simulink model "S_MPPT_ALGS_PIL_SIM_V1"  (R2017a)
settings: Solver=VariableStepAuto  StartTime=0.0  StopTime=5  FixedStep=1e-6  MaxStep=1e-4  RelTol=1e-3
values from neighbouring files (symbols this model uses):
  Alpha1 = 2*Zeta_obs*wn_obs    (= 2)    [M_MPPT_ALGS_PIL_SIM_V1.m]
  Alpha2 = wn_obs    (= 1)    [M_MPPT_ALGS_PIL_SIM_V1.m]
  Cdc = Cdc    (= 0.00047)    [M_MPPT_ALGS_PIL_SIM_V1.m]
  Cpv = Cpv    (= 8e-05)    [M_MPPT_ALGS_PIL_SIM_V1.m]
  Epsilon = Ep_cont/Ts1    [M_MPPT_ALGS_PIL_SIM_V1.m]
  ESRCdc = ESRCdc    (= 0.2)    [M_MPPT_ALGS_PIL_SIM_V1.m]
  ESRCpv = ESRCpv    (= 0.2)    [M_MPPT_ALGS_PIL_SIM_V1.m]
  Fred = fs    (= 60)    [M_MPPT_ALGS_PIL_SIM_V1.m]
  fs = 60    [M_MPPT_ALGS_PIL_SIM_V1.m]
  G_STC = 1000    [M_MPPT_ALGS_PIL_SIM_V1.m]
  Icc_calc = In/(5/100)    [M_MPPT_ALGS_PIL_SIM_V1.m]
  impp_STC = 15.72/2    (= 7.86)    [M_MPPT_ALGS_PIL_SIM_V1.m]
  K1 = Kt_acker_d    [M_MPPT_ALGS_PIL_SIM_V1.m]
  K1y2md = Kmd(1:end-1)    [M_MPPT_ALGS_PIL_SIM_V1.m]
  Kdpwm = 1/Ucmax    (= 1.52590218967e-05)    [M_MPPT_ALGS_PIL_SIM_V1.m]
  KI1 = Kp1/Ti1*Ts1    (= 1900)    [M_MPPT_ALGS_PIL_SIM_V1.m]
  KI2 = Ki2*Ts4    [M_MPPT_ALGS_PIL_SIM_V1.m]
  KI4 = Ki4*Ts4    [M_MPPT_ALGS_PIL_SIM_V1.m]
  KI5 = Ki5*Ts_inv    (= 0.17765287922)    [M_MPPT_ALGS_PIL_SIM_V1.m]
  Kimd = -Kmd(end)    [M_MPPT_ALGS_PIL_SIM_V1.m]
  KP1 = Kp1-KI1/2    (= 21850)    [M_MPPT_ALGS_PIL_SIM_V1.m]
  KP2 = Kp2-KI2/2    [M_MPPT_ALGS_PIL_SIM_V1.m]
  KP4 = Kp4-KI4/2    [M_MPPT_ALGS_PIL_SIM_V1.m]
  KP5 = Kp5*Ts_inv-KI5/2    (= -0.0874937760062)    [M_MPPT_ALGS_PIL_SIM_V1.m]
  L = L    (= 0.1)    [M_MPPT_ALGS_PIL_SIM_V1.m]
  Linv = 0.03    [M_MPPT_ALGS_PIL_SIM_V1.m]
  Npar = No_Cadenas_Paralelo    (= 2)    [M_MPPT_ALGS_PIL_SIM_V1.m]
  Rinv = 0.0417    [M_MPPT_ALGS_PIL_SIM_V1.m]
  RL = RL    (= 0.3)    [M_MPPT_ALGS_PIL_SIM_V1.m]
  S = 10e3*3/2    (= 15000)    [M_MPPT_ALGS_PIL_SIM_V1.m]
  Ts = Ts1    (= 0.0002)    [M_MPPT_ALGS_PIL_SIM_V1.m]
  Ts1 = 1/Fs    (= 0.0002)    [M_MPPT_ALGS_PIL_SIM_V1.m]
  Ts4 = 1/(4*Fc)    (= 0.000125)    [M_MPPT_ALGS_PIL_SIM_V1.m]
  Ts_inv = 1/(100*Fc)    (= 5e-06)    [M_MPPT_ALGS_PIL_SIM_V1.m]
  Ucmax = (2^b-1)    (= 65535)    [M_MPPT_ALGS_PIL_SIM_V1.m]
  vdc = 1000    [M_MPPT_ALGS_PIL_SIM_V1.m]
  vdc_ref = vdc    (= 1000)    [M_MPPT_ALGS_PIL_SIM_V1.m]
  Vf = VL/sqrt(3)    [M_MPPT_ALGS_PIL_SIM_V1.m]
  VL = (381.051/2)    (= 190.5255)    [M_MPPT_ALGS_PIL_SIM_V1.m]
undefined symbols (not defined in the file or in its folder): DiscIntNeverNeededParam
undefined symbols (not defined in the file): Fs
libraries: powerlib x15, powerlib_meascontrol x12, dsparch4 x3, re_lib x1
(part 1 of 2)
settings Model: ExtModeTrigDuration=10  Creator=dricl  LastModifiedBy=dricl
settings OptimizationCC: PassReuseOutputArgsAs=Individual arguments  MaxStackSize=2560
settings DebuggingCC: ParameterTunabilityLossMsg=error
settings HardwareCC: ProdBitPerPointer=32  ProdBitPerSizeT=32  ProdBitPerPtrDiffT=32  ProdLargestAtomicInteger=Long  ProdLargestAtomicFloat=Double  ProdWordSize=32  ProdLongLongMode=on  ProdHWDeviceType=ARM Compatible->ARM Cortex
settings SFSimCC: MATLABDynamicMemAlloc=off
settings RTWCC: SystemTargetFile=ert.tlc  HardwareBoard=TI Concerto F28M35x (ARM Cortex-M3)  TLCOptions=-aInlineSetEventsForThisBaseRateFcn=TLC_FALSE -aSuppressMultiTaskScheduler=TLC_FALSE -aRateBasedStepFcn=1  TemplateMakefile=ert_default_tmf  Description=Embedded Coder  GenerateReport=on  Toolchain=Texas Instruments Code Composer Studio v6 (ARM)  IncludeHyperlinkInReport=on  LaunchReport=on  CreateSILPILBlock=PIL  GenerateTraceInfo=on  GenerateTraceReport=on  GenerateTraceReportSl=on  GenerateTraceReportSf=on  GenerateTraceReportEml=on
settings CodeAppCC: ForceParamTrailComments=on  IgnoreCustomStorageClasses=off  OperatorAnnotations=on  SimulinkDataObjDesc=on  SFDataObjDesc=on  MATLABFcnDesc=on  InsertBlockDesc=on  MATLABSourceComments=on

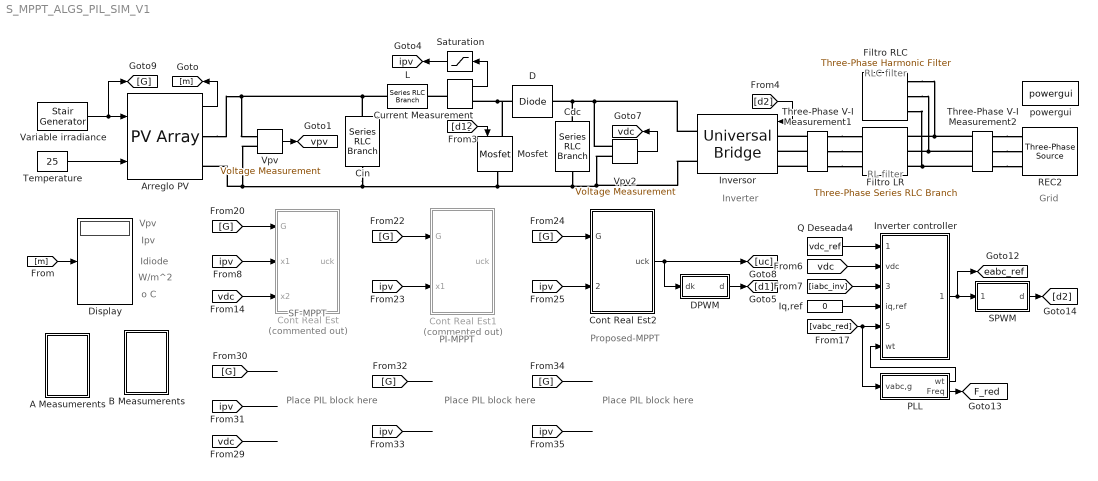
== system S_MPPT_ALGS_PIL_SIM_V1 ==
  note: Grid
  note: W/m^2
  note: Idiode
  note: Vpv
  note: RLC filter
  note: Ipv
  note: SF-MPPT
  note: PI-MPPT
  note: o C
  note: Proposed-MPPT
  note: RL filter
  note: Inverter
  note: Place PIL
      | block here
  note: Place PIL
      | block here
  note: Place PIL
      | block here
  " Variable irradiance" : powerlib_meascontrol/Pulse & Signal Generators/Stair Generator  t=[0, 0.1, 0.3, 0.5, 0.7, 0.8, 0.9, 1.0, 1.1, 1.2, 1.3, 1.4, 1.5, 1.6, 1.7, 1.8, 1.9, 2.0, 2.1, 2.2, 2.3, 2.4, 2.5, 2.6, 2.7, 2.8, 2.9, 3.0, 3.1, 3.2, 3.3, 3.4, 3.5, 3.6, 3.7, 3.8, 3.9, 4.0, 4.1, 4.2, 4.3, 4.4, 4.5, 4.6, 4.7, 4.8, 4.9, 5.0]  e=[0, 1000, 400, 900, 607.1, 607.1, 652.7, 685.8, 715.6, 742.3, 765.3, 795, 812, 840, 839, 893, 596.3, 420.8, 1037, 974, 948, 921, 970, 985, 991, 700, 1004, 997, 993, 1001, 998, 1033, 656.5, 1027, 954, 938, 937, 906, 705.4, 860, 773, 670.6, 450.3, 409.6, 682.2, 639.9, 601, 415.5]  Ts=0
      settings: SourceProductName=Simscape Power Systems
  A Measumerents : Subsystem
  Arreglo PV : re_lib/Solar/PV Array  Npar=No_Cadenas_Paralelo  Nser=No_Modulos_PorCadena  PlotType=array @ 25 deg.C & specified irradiances  S_vec=[1037]  Temp_C_vec="[ 45 25  0]"  ModuleName=Canadian Solar CS6X-280P  PlotWhenSelected=off  Pm=279.816  Ncell=72  Voc=44.2  Isc=8.42  Vm=35.6  Im=7.86  beta_Voc_pc=-0.39  alpha_Isc_pc=0.06  beta_Voc=-0.17238  alpha_Isc=0.005052  IL=8.4417  I0=7.7188e-10  nI=1.0345  Rsh=300.2269  Rs=0.38773  BAL=off  Tc=1e-6  Tfilter=5e-5
  B Measumerents : Subsystem
  Cdc : powerlib/Elements/Series RLC Branch  LConnTagsString=__new0  RConnTagsString=__new0  BranchType=RC  Resistance=ESRCdc  Inductance=1e-3  SetiL0=off  InitialCurrent=0  Capacitance=Cdc  Setx0=on  InitialVoltage=vdc_ref  Measurements=None
  Cin : powerlib/Elements/Series RLC Branch  LConnTagsString=__new0  RConnTagsString=__new0  BranchType=RC  Resistance=ESRCpv  Inductance=1e-3  SetiL0=off  InitialCurrent=0  Capacitance=Cpv  Setx0=off  InitialVoltage=640.8  Measurements=None
  Cont Real Est : Subsystem  Commented=on
  Cont Real Est1 : Subsystem  Commented=on
  Cont Real Est2 : Subsystem
  Current Measurement2 : powerlib/Measurements/Current Measurement  PhasorSimulation=off  OutputType=Complex  PSBequivalent=0
  D : powerlib/Power Electronics/Diode  Ron=Rondiode  Lon=0  Vf=Vfdiode  IC=0  UseSnubber=0  Rs=500  Cs=250e-9  Measurements=off
  DPWM : Subsystem  AncestorBlock=plecslib_extras2/Modulators/Symmetrical PWM  mask(Symmetrical PWM){sampling=Natural (carrier starts with 0), fc=Fs, offset=0, input_limits=[0 Ucmax], output_values=[0 1]}
      mask prompts: fc "Carrier frequency (Hz):"; offset "Carrier offset (p.u.):"; input_limits "Input limits [min max]:"; output_values "Output values [off on]:"
      mask help: PWM generator with a symmetrical triangular carrier. If the input is a vector, the output is also a vector of the same width.
      mask init:
      | if numel(fc)>1 || fc<=0,
      |   error('Carrier frequency must be a positive scalar.');
      | end
      | if numel(offset)>1 || offset<0 || offset>=1,
      |   error('Carrier offset must be a scalar in the range [0; 1/fc[.');
      | end
      | if sampling == 1,
      |   offset = mod(offset+.75, 1);
      | end
      | 
      | si = [.5 mod(offset, .5)]/fc;
      mask Help: eval('plecs(''help'', ''symmetricalpwm.html'')')
      mask TypeOptions sampling: Natural (carrier starts with 0) | Natural (carrier starts with 1) | Regular (double edge) | Regular (single edge)
  Display : Display
  Filtro LR : powerlib/Elements/Three-Phase Series RLC Branch  LConnTagsString=A|B|C  RConnTagsString=A|B|C  BranchType=RL  Resistance=Rinv  Inductance=Linv  Capacitance=1e-6  Measurements=None
  Filtro RLC : powerlib/Elements/Three-Phase Harmonic Filter  LConnTagsString=A|B|C  FilterType=Single-tuned  FilterConnection=Y (grounded)  ParNom=[VL fs]  Qc=S*0.001  Fr=[31.42*60]  Frd=[40*fs 80*fs]  Q=5  Measurements=None
      settings: AttributesFormatString=\n  SourceProductName=Simscape Power Systems  SourceProductBaseCode=PS
  Inversor : powerlib/Power Electronics/Universal Bridge  Arms=3  SnubberResistance=1e5  SnubberCapacitance=inf  Device=IGBT / Diodes  Ron=1e-3  Lon=0  ForwardVoltages="[  0  0  ]"  ForwardVoltage=0  GTOparameters=[ 10e-6 , 20e-6 ]  IGBTparameters=[ 1e-6 , 2e-6 ]  Measurements=None  Measurements_2=None  converterType=Rectifier
  Inverter controller : Subsystem
  Iq,ref : Constant  Value=0  SampleTime=Ts4
  L : powerlib/Elements/Series RLC Branch  LConnTagsString=__new0  RConnTagsString=__new0  BranchType=RL  Resistance=RL  Inductance=L  SetiL0=off  InitialCurrent=0  Capacitance=1e-6  Setx0=off  InitialVoltage=0  Measurements=None
  Mosfet : powerlib/Power Electronics/Mosfet  Ron=Ronfet  Lon=0  Rd=0  Vfd=0  IC=0  Rs=1e5  Cs=inf  Measurements=off
  PLL : Subsystem
  Q Deseada4 : Constant  Value=vdc_ref  SampleTime=Ts4
  REC2 : powerlib/Electrical Sources/Three-Phase Source  InternalConnection=Yg  VoltagePhases=on  Voltage=VL  PhaseAngle=0  Voltage_phases=[VL/sqrt(3) VL/sqrt(3) VL/sqrt(3)]  PhaseAngles_phases=[0 -120 +120]  Frequency=Fred  NonIdealSource=on  SpecifyImpedance=on  Resistance=25e3^2/10e6/5  Inductance=25e3^2/10e6/377  ShortCircuitLevel=Icc_calc*2  BaseVoltage=VL  XRratio=7  BusType=swing  Pref=-500e3  Qref=0  Prefabc=[10e3, 10e3, 10e3]  Qrefabc=[0, 0, 0]  Qmin=-inf  Qmax=inf
  SPWM : Subsystem
  Saturation : Saturate  UpperLimit=inf  LowerLimit=0
  Temperature : Constant  Value=25
  Three-Phase V-I Measurement1 : powerlib/Measurements/Three-Phase V-I Measurement  VoltageMeasurement=phase-to-ground  SetLabelV=on  LabelV=vabc_inv  Vpu=off  VpuLL=off  CurrentMeasurement=yes  SetLabelI=on  LabelI=iabc_inv  Ipu=off  Pbase=100e6  Vbase=500e3  OutputType=Complex  PhasorSimulation=off  PSBequivalent=0
  Three-Phase V-I Measurement2 : powerlib/Measurements/Three-Phase V-I Measurement  VoltageMeasurement=phase-to-ground  SetLabelV=on  LabelV=vabc_red  Vpu=off  VpuLL=off  CurrentMeasurement=yes  SetLabelI=on  LabelI=iabc_red  Ipu=off  Pbase=100e6  Vbase=500e3  OutputType=Complex  PhasorSimulation=off  PSBequivalent=0
  Vpv : powerlib/Measurements/Voltage Measurement  PhasorSimulation=off  OutputType=Complex  PSBequivalent=0
  Vpv2 : powerlib/Measurements/Voltage Measurement  PhasorSimulation=off  OutputType=Complex  PSBequivalent=0
  powergui : powerlib/powergui  Priority=1  SimulationMode=Continuous  SampleTime=1e-6  frequency=60  Iterations=50  frequencyindice=0  Pbase=100e6  ErrMax=1e-4  UnitsV=kV  UnitsW=MW  buscounter=0  FunctionMessages=off  echomessages=off  EnableUseOfTLC=off  CurrentSourceSwitches=off  DisableSnubberDevices=off  DisableRonSwitches=off  DisableVfSwitches=off  DisplayEquations=off  SolverType=Tustin/Backward Euler (TBE)  Interpol=off  ExternalGateDelay=off  methode=off  Ts=100  x0status=blocks  SPID=on  SwTol=0  HookPort=off  RestoreLinks=warning  ResistiveCurrentMeasurement=off  Frange=[0:2:500]  Ylog=off  Xlog=on  ShowGrid=off  save=off  variable=ZData  structure=0  ZoomFFT=off  StartTime=0.0  cycles=1  DisplayStyle=1  fundamental=60  FreqAxis=off  MaxFrequency=1000  frequencyindicesteady=1  RmsSteady=1  display=off
  tag scope: F_red=global, eabc_ref=global, ipv=global, vdc=global, vpv=global
  wires:
  [iabc_inv] -> Inverter controller/3(iabc,inv)
  Iq,ref/1 -> Inverter controller/4(iq,ref)
  Vpv2/1 -> [vdc]
  Q Deseada4/1 -> Inverter controller/1(vdc,ref)
  PLL/2(Freq) -> [F_red]
  SPWM/1(d) -> [d2]
  DPWM/1(d) -> [d1]
  Saturation/1 -> [ipv]
  Temperature/1 -> Arreglo PV/2
  [vdc] -> Inverter controller/2(vdc)
  PLL/1(wt) -> Inverter controller/6(wt)
  [vabc_red] -> PLL/1(vabc,g), Inverter controller/5(vabc,red)
  [d2] -> Inversor/1
  Vpv/1 -> [vpv]
  Inverter controller/1(eabc,ref) -> SPWM/1(eabc,ref), [eabc_ref]
  [d1] -> Mosfet/1
  Current Measurement2/1 -> Saturation/1
  [m] -> Display/1
  Arreglo PV/1 -> [m]
  [G] -> Cont Real Est1/1(G)
  [ipv] -> Cont Real Est1/2(x1)
  [ipv] -> Cont Real Est2/2(x1 = ipv)
  [ipv] -> Cont Real Est/2(x1)
  [vdc] -> Cont Real Est/3(x2)
  [G] -> Cont Real Est/1(G)
  " Variable irradiance"/1 -> [G], Arreglo PV/1
  [G] -> Cont Real Est2/1(G)
  [G] -> ?
  [ipv] -> ?
  [G] -> ?
  [ipv] -> ?
  [G] -> ?
  [ipv] -> ?
  [vdc] -> ?
  Cont Real Est2/1(uck) -> DPWM/1(dk), [uc]
  connections:
  Arreglo PV/RConn1 -- L/LConn1 -- Cin/LConn1 -- Vpv/LConn1
  Filtro RLC/LConn1 -- Filtro LR/RConn1 -- Three-Phase V-I Measurement2/LConn1
  Three-Phase V-I Measurement2/RConn1 -- REC2/RConn1
  Cdc/RConn1 -- Inversor/RConn2 -- Vpv2/LConn2 -- Vpv/LConn2 -- Arreglo PV/RConn2 -- Cin/RConn1 -- Mosfet/RConn1
  Filtro RLC/LConn2 -- Filtro LR/RConn2 -- Three-Phase V-I Measurement2/LConn2
  Three-Phase V-I Measurement2/RConn2 -- REC2/RConn2
  D/RConn1 -- Cdc/LConn1 -- Vpv2/LConn1 -- Inversor/RConn1
  Filtro RLC/LConn3 -- Filtro LR/RConn3 -- Three-Phase V-I Measurement2/LConn3
  Three-Phase V-I Measurement2/RConn3 -- REC2/RConn3
  Current Measurement2/RConn1 -- D/LConn1 -- Mosfet/LConn1
  Three-Phase V-I Measurement1/RConn1 -- Filtro LR/LConn1
  Three-Phase V-I Measurement1/RConn2 -- Filtro LR/LConn2
  Three-Phase V-I Measurement1/RConn3 -- Filtro LR/LConn3
  Three-Phase V-I Measurement1/LConn2 -- Inversor/LConn2
  Current Measurement2/LConn1 -- L/RConn1
  Three-Phase V-I Measurement1/LConn1 -- Inversor/LConn1
  Three-Phase V-I Measurement1/LConn3 -- Inversor/LConn3

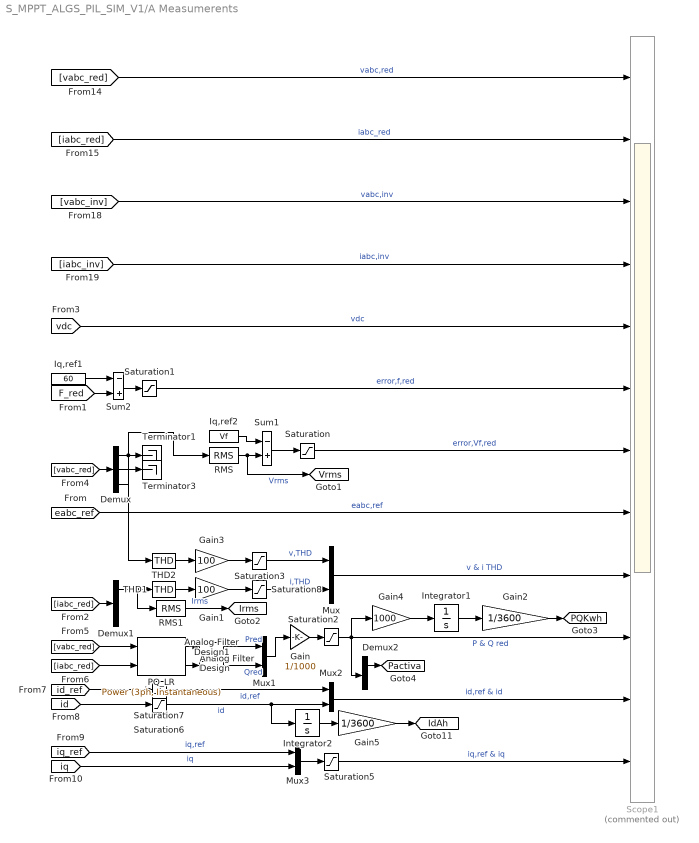
== system S_MPPT_ALGS_PIL_SIM_V1/A Measumerents ==
  Analog Filter Design : dsparch4/Analog Filter Design  method=Butterworth  filttype=Lowpass  N=8  Wlo=4000  Whi=80  Rp=2  Rs=40
  Analog Filter Design1 : dsparch4/Analog Filter Design  method=Butterworth  filttype=Lowpass  N=8  Wlo=4000  Whi=80  Rp=2  Rs=40
  Demux : Demux  Outputs=3
  Demux1 : Demux  Outputs=3
  Demux2 : Demux  Outputs=2
  Gain : Gain  Gain=1/1000
  Gain1 : Gain  Gain=100
  Gain2 : Gain  Gain=1/3600
  Gain3 : Gain  Gain=100
  Gain4 : Gain  Gain=1000
  Gain5 : Gain  Gain=1/3600
  Integrator1 : Integrator  ZeroCross=off
  Integrator2 : Integrator  ZeroCross=off
  Iq,ref1 : Constant  Value=60  SampleTime=Ts4
  Iq,ref2 : Constant  Value=Vf  SampleTime=Ts4
  Mux{,1..3} (4 alike) : Mux  Inputs=2
  PQ_LR : powerlib_meascontrol/Measurements/Power (3ph, Instantaneous)
      settings: SourceProductName=Simscape Power Systems
  RMS : powerlib_meascontrol/Measurements/RMS  TrueRMS=on  Freq=60  RMSInit=0  Ts=0
  RMS1 : powerlib_meascontrol/Measurements/RMS  TrueRMS=on  Freq=60  RMSInit=0  Ts=0
  Saturation : Saturate  UpperLimit=5.5  LowerLimit=-5.5
  Saturation1 : Saturate  UpperLimit=1  LowerLimit=-1
  Saturation2 : Saturate  UpperLimit=20  LowerLimit=0
  Saturation3 : Saturate  UpperLimit=20  LowerLimit=0
  Saturation5 : Saturate  UpperLimit=100  LowerLimit=0
  Saturation6 : Saturate  UpperLimit=inf  LowerLimit=0
  Saturation7 : Saturate  UpperLimit=inf  LowerLimit=0
  Saturation8 : Saturate  UpperLimit=20  LowerLimit=0
  Scope1 : Scope  Commented=on  NumInputPorts=12
  Sum1 : Sum  Inputs=-+
  Sum2 : Sum  Inputs=-+
  THD1 : powerlib_meascontrol/Measurements/THD  Freq=60  Ts=0
  THD2 : powerlib_meascontrol/Measurements/THD  Freq=60  Ts=0
  Terminator1 : Terminator
  Terminator3 : Terminator
  tag scope: IdAh=global, Irms=global, PQKwh=global, Pactiva=global, Vrms=global
  wires:
  Saturation/1 -> Scope1/7  "error,Vf,red"
  [vabc_red] -> Scope1/1  "vabc,red"
  [eabc_ref] -> Scope1/8  "eabc,ref"
  [iabc_red] -> Scope1/2  "iabc_red"
  Demux/1 -> THD2/1, RMS/1
  [vdc] -> Scope1/5  "vdc"
  [iabc_inv] -> Scope1/4  "iabc,inv"
  [vabc_inv] -> Scope1/3  "vabc,inv"
  Sum1/1 -> Saturation/1
  RMS/1 -> [Vrms], Sum1/2  "Vrms"
  Demux/2 -> Terminator3/1
  Demux/3 -> Terminator1/1
  [vabc_red] -> Demux/1
  [F_red] -> Sum2/2
  Iq,ref2/1 -> Sum1/1
  Iq,ref1/1 -> Sum2/1
  Saturation1/1 -> Scope1/6  "error,f,red"
  Sum2/1 -> Saturation1/1
  [iabc_red] -> Demux1/1
  Demux1/1 -> RMS1/1, THD1/1
  THD2/1 -> Gain3/1
  THD1/1 -> Gain1/1
  Mux/1 -> Scope1/9  "v & i THD"
  [vabc_red] -> PQ_LR/1
  [iabc_red] -> PQ_LR/2
  PQ_LR/1 -> Analog Filter Design/1
  Analog Filter Design/1 -> Mux1/1  "Pred"
  PQ_LR/2 -> Analog Filter Design1/1
  Analog Filter Design1/1 -> Mux1/2  "Qred"
  Saturation2/1 -> Demux2/1, Gain4/1, Scope1/10  "P & Q red"
  Gain/1 -> Saturation2/1
  Mux1/1 -> Gain/1
  Mux3/1 -> Saturation5/1
  [iq] -> Mux3/2  "iq"
  [id] -> Saturation6/1
  [iq_ref] -> Mux3/1  "iq,ref"
  [id_ref] -> Saturation7/1
  Mux2/1 -> Scope1/11  "id,ref & id"
  Saturation5/1 -> Scope1/12  "iq,ref & iq"
  RMS1/1 -> [Irms]  "Irms"
  Saturation6/1 -> Integrator2/1, Mux2/2  "id"
  Saturation7/1 -> Mux2/1  "id,ref"
  Gain3/1 -> Saturation3/1
  Saturation3/1 -> Mux/1  "v,THD"
  Saturation8/1 -> Mux/2  "i,THD"
  Gain1/1 -> Saturation8/1
  Integrator2/1 -> Gain5/1
  Integrator1/1 -> Gain2/1
  Demux2/1 -> [Pactiva]
  Gain2/1 -> [PQKwh]
  Gain4/1 -> Integrator1/1
  Gain5/1 -> [IdAh]

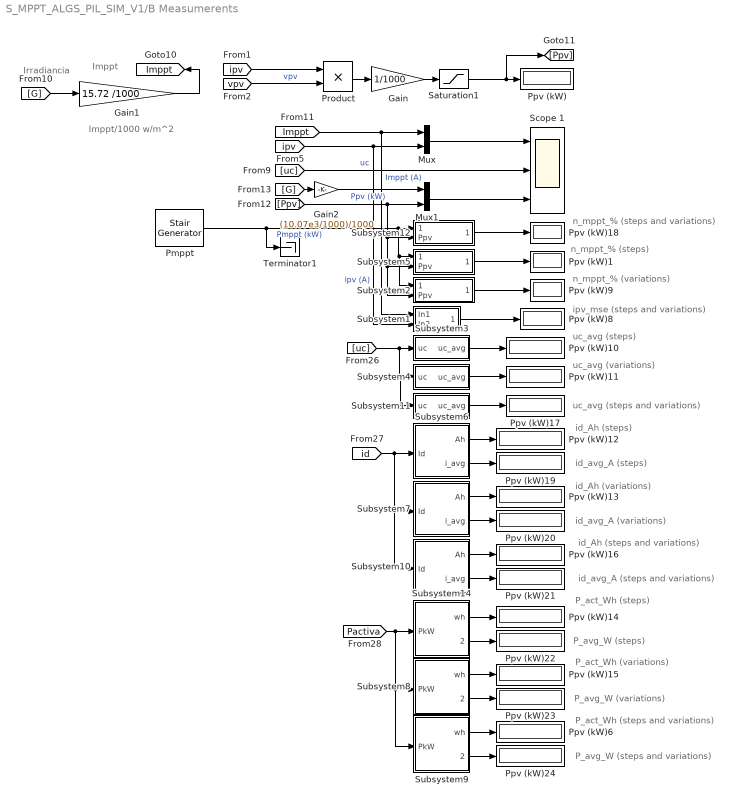
== system S_MPPT_ALGS_PIL_SIM_V1/B Measumerents ==
  note: P_act_Wh (steps)
  note: ipv_mse (steps and variations)
  note: n_mppt_% (steps)
  note: uc_avg (steps)
  note: n_mppt_% (variations)
  note: uc_avg (variations)
  note: id_Ah (steps)
  note: id_Ah (variations)
  note: P_act_Wh (variations)
  note: n_mppt_% (steps and variations)
  note: P_act_Wh (steps and variations)
  note: id_Ah (steps and variations)
  note: uc_avg (steps and variations)
  note: id_avg_A (steps)
  note: id_avg_A (variations)
  note: id_avg_A (steps and variations)
  note: P_avg_W (steps)
  note: P_avg_W (variations)
  note: P_avg_W (steps and variations)
  note: Irradiancia
  note: Imppt
  note: Imppt/1000 w/m^2
  Gain : Gain  Gain=1/1000
  Gain1 : Gain  Gain=15.72 /1000
  Gain2 : Gain  Gain=(10.07e3/1000)/1000
  Mux : Mux  Inputs=2
  Mux1 : Mux  Inputs=2
  Pmppt : powerlib_meascontrol/Pulse & Signal Generators/Stair Generator  t=[0, 0.1, 0.3, 0.5, 0.7, 0.8, 0.9, 1.0, 1.1, 1.2, 1.3, 1.4, 1.5, 1.6, 1.7, 1.8, 1.9, 2.0, 2.1, 2.2, 2.3, 2.4, 2.5, 2.6, 2.7, 2.8, 2.9, 3.0, 3.1, 3.2, 3.3, 3.4, 3.5, 3.6, 3.7, 3.8, 3.9, 4.0, 4.1, 4.2, 4.3, 4.4, 4.5, 4.6, 4.7, 4.8, 4.9, 5.0]  e=[0, 10.07, 4.040, 9.089, 6.158, 6.158, 6.662, 6.954, 7.254, 7.522, 7.752, 8.049, 8.218, 8.497, 8.487, 9.020, 6.048, 4.254, 10.43, 9.816, 9.561, 9.294, 9.777, 9.924, 9.982, 7.097, 10.11, 10.04, 10.00, 10.08, 10.05, 10.39, 6.658, 10.33, 9.620, 9.462, 9.453, 9.147, 7.151, 8.695, 7.829, 6.801, 4.557, 4.138, 6.918, 6.490, 6.096, 4.199]  Ts=0
      settings: SourceProductName=Simscape Power Systems
  Ppv (kW){,1,6,8..24} (20 alike) : Display
  Product : Product
  Saturation1 : Saturate  UpperLimit=inf  LowerLimit=0
  Scope 1 : Scope  NumInputPorts=3
  Subsystem1 : Subsystem
  Subsystem10 : Subsystem
  Subsystem11 : Subsystem
  Subsystem12 : Subsystem
  Subsystem14 : Subsystem
  Subsystem2 : Subsystem
  Subsystem3 : Subsystem
  Subsystem4 : Subsystem
  Subsystem5 : Subsystem
  Subsystem6 : Subsystem
  Subsystem7 : Subsystem
  Subsystem8 : Subsystem
  Subsystem9 : Subsystem
  Terminator1 : Terminator
  tag scope: Imppt=global
  wires:
  [Imppt] -> Subsystem1/1(In1), Mux/1  "Imppt (A)"
  [G] -> Gain2/1
  Saturation1/1 -> [Ppv], Ppv (kW)/1
  [uc] -> Subsystem11/1(uc), Subsystem4/1(uc), Subsystem3/1(uc)
  [vpv] -> Product/2  "vpv"
  Mux1/1 -> Scope 1/3
  [ipv] -> Product/1
  Subsystem1/1(Out1) -> Ppv (kW)8/1
  Subsystem12/1(n_mppt) -> Ppv (kW)18/1
  Gain2/1 -> Mux1/1
  [ipv] -> Subsystem1/2(In2), Mux/2  "ipv (A)"
  Gain/1 -> Saturation1/1
  Product/1 -> Gain/1
  Mux/1 -> Scope 1/1
  Subsystem3/1(uc_avg) -> Ppv (kW)10/1
  Subsystem2/1(nmppt) -> Ppv (kW)9/1
  Subsystem4/1(uc_avg) -> Ppv (kW)11/1
  Subsystem11/1(uc_avg) -> Ppv (kW)17/1
  [id] -> Subsystem10/1(Id), Subsystem7/1(Id), Subsystem6/1(Id)
  Subsystem6/2(i_avg) -> Ppv (kW)19/1
  Subsystem7/1(Ah) -> Ppv (kW)13/1
  Subsystem10/1(Ah) -> Ppv (kW)16/1
  Subsystem5/1(nmppt) -> Ppv (kW)1/1
  Subsystem6/1(Ah) -> Ppv (kW)12/1
  [uc] -> Scope 1/2  "uc"
  Subsystem7/2(i_avg) -> Ppv (kW)20/1
  Pmppt/1 -> Terminator1/1, Subsystem2/1(Pmpp), Subsystem5/1(Pmpp), Subsystem12/1(Pmpp)  "Pmppt (kW)"
  [Pactiva] -> Subsystem9/1(PkW), Subsystem8/1(PkW), Subsystem14/1(PkW)
  Subsystem10/2(i_avg) -> Ppv (kW)21/1
  Subsystem14/1(wh) -> Ppv (kW)14/1
  Subsystem8/1(wh) -> Ppv (kW)15/1
  Subsystem8/2(Pw_avg) -> Ppv (kW)23/1
  Subsystem9/2(Pw_avg) -> Ppv (kW)24/1
  [Ppv] -> Mux1/2, Subsystem12/2(Ppv), Subsystem2/2(Ppv), Subsystem5/2(Ppv)  "Ppv (kW)"
  Subsystem9/1(wh) -> Ppv (kW)6/1
  Subsystem14/2(Pw_avg) -> Ppv (kW)22/1
  Gain1/1 -> [Imppt]
  [G] -> Gain1/1

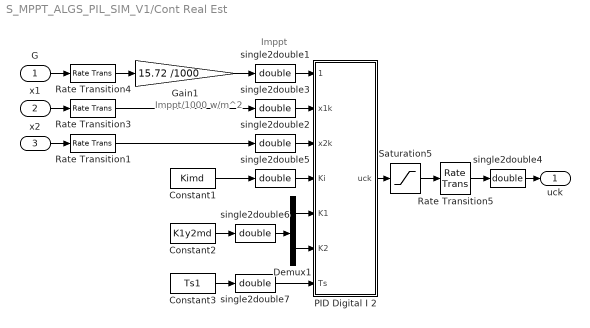
== system S_MPPT_ALGS_PIL_SIM_V1/Cont Real Est ==
  note: Imppt/1000 w/m^2
  note: Imppt
  G : Inport
  x1 : Inport  Port=2
  x2 : Inport  Port=3
  Constant1 : Constant  Value=Kimd  SampleTime=Ts1
  Constant2 : Constant  Value=K1y2md  SampleTime=Ts1
  Constant3 : Constant  Value=Ts1  SampleTime=Ts1
  Demux1 : Demux  Outputs=2
  Gain1 : Gain  Gain=15.72 /1000
  PID Digital I 2 : MATLAB Function  TreatAsAtomicUnit=on
  Rate Transition{1,3..5} (4 alike) : RateTransition  Deterministic=off  OutPortSampleTime=Ts1
  Saturation5 : Saturate  UpperLimit=Ucmax  LowerLimit=0
  single2double{1..7} (7 alike) : DataTypeConversion  OutDataTypeStr=double
  uck : Outport
  wires:
  Constant3/1 -> single2double7/1
  PID Digital I 2/1(uck) -> Saturation5/1
  Constant1/1 -> single2double5/1
  Demux1/1 -> PID Digital I 2/5(K1)
  Demux1/2 -> PID Digital I 2/6(K2)
  Rate Transition3/1 -> single2double3/1
  Rate Transition5/1 -> single2double4/1
  single2double1/1 -> PID Digital I 2/1(x1k_Ref)
  single2double3/1 -> PID Digital I 2/2(x1k)
  Rate Transition1/1 -> single2double2/1
  single2double2/1 -> PID Digital I 2/3(x2k)
  x2/1 -> Rate Transition1/1
  x1/1 -> Rate Transition3/1
  G/1 -> Rate Transition4/1
  single2double4/1 -> uck/1
  Saturation5/1 -> Rate Transition5/1
  single2double5/1 -> PID Digital I 2/4(Ki)
  Constant2/1 -> single2double6/1
  single2double6/1 -> Demux1/1
  single2double7/1 -> PID Digital I 2/7(Ts)
  Gain1/1 -> single2double1/1
  Rate Transition4/1 -> Gain1/1

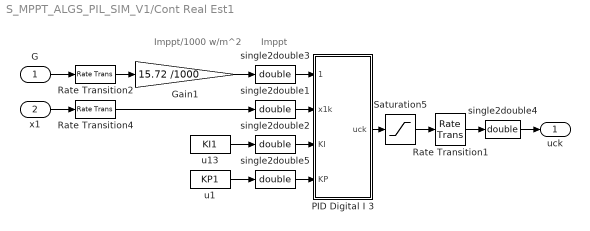
== system S_MPPT_ALGS_PIL_SIM_V1/Cont Real Est1 ==
  note: Imppt
  note: Imppt/1000 w/m^2
  G : Inport
  x1 : Inport  Port=2
  Gain1 : Gain  Gain=15.72 /1000
  PID Digital I 3 : MATLAB Function  TreatAsAtomicUnit=on
  Rate Transition1 : RateTransition  Deterministic=off  OutPortSampleTime=Ts1
  Rate Transition2 : RateTransition  Deterministic=off  OutPortSampleTime=Ts1
  Rate Transition4 : RateTransition  Deterministic=off  OutPortSampleTime=Ts1
  Saturation5 : Saturate  UpperLimit=Ucmax  LowerLimit=0
  single2double{1..5} (5 alike) : DataTypeConversion  OutDataTypeStr=double
  u1 : Constant  Value=KP1  SampleTime=Ts1
  u13 : Constant  Value=KI1  SampleTime=Ts1
  uck : Outport
  wires:
  u1/1 -> single2double5/1
  u13/1 -> single2double2/1
  PID Digital I 3/1(uck) -> Saturation5/1
  Rate Transition4/1 -> single2double1/1
  single2double3/1 -> PID Digital I 3/1(x1k_ref)
  single2double1/1 -> PID Digital I 3/2(x1k)
  x1/1 -> Rate Transition4/1
  Rate Transition1/1 -> single2double4/1
  single2double4/1 -> uck/1
  Saturation5/1 -> Rate Transition1/1
  single2double2/1 -> PID Digital I 3/3(KI)
  single2double5/1 -> PID Digital I 3/4(KP)
  G/1 -> Rate Transition2/1
  Rate Transition2/1 -> Gain1/1
  Gain1/1 -> single2double3/1

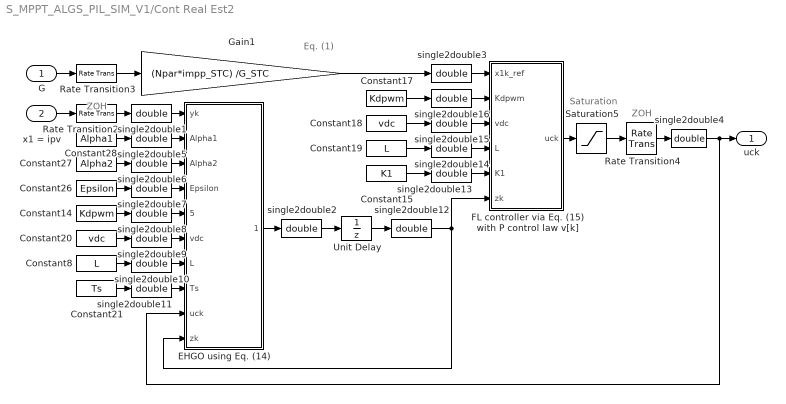
== system S_MPPT_ALGS_PIL_SIM_V1/Cont Real Est2 ==
  note: ZOH
  note: Saturation
  note: Eq. (1)
  note: ZOH
  G : Inport
  x1 = ipv : Inport  Port=2
  Constant14 : Constant  Value=Kdpwm  SampleTime=Ts1
  Constant15 : Constant  Value=K1  SampleTime=Ts1
  Constant17 : Constant  Value=Kdpwm  SampleTime=Ts1
  Constant18 : Constant  Value=vdc  SampleTime=Ts1
  Constant19 : Constant  Value=L  SampleTime=Ts1
  Constant20 : Constant  Value=vdc  SampleTime=Ts1
  Constant21 : Constant  Value=Ts  SampleTime=Ts1
  Constant26 : Constant  Value=Epsilon  SampleTime=Ts1
  Constant27 : Constant  Value=Alpha2  SampleTime=Ts1
  Constant28 : Constant  Value=Alpha1  SampleTime=Ts1
  Constant8 : Constant  Value=L  SampleTime=Ts1
  EHGO using Eq. (14) : MATLAB Function  TreatAsAtomicUnit=on
  FL controller via Eq. (15) with P control law v[k] : MATLAB Function  TreatAsAtomicUnit=on
  Gain1 : Gain  Gain=(Npar*impp_STC) /G_STC
  Rate Transition2 : RateTransition  Deterministic=off  OutPortSampleTime=Ts1
  Rate Transition3 : RateTransition  Deterministic=off  OutPortSampleTime=Ts1
  Rate Transition4 : RateTransition  Deterministic=off  OutPortSampleTime=Ts1
  Saturation5 : Saturate  UpperLimit=Ucmax  LowerLimit=0
  Unit Delay : UnitDelay  SampleTime=Ts1
  single2double{1..16} (16 alike) : DataTypeConversion  OutDataTypeStr=double
  uck : Outport
  wires:
  x1 = ipv/1 -> Rate Transition2/1
  Rate Transition2/1 -> single2double1/1
  Gain1/1 -> single2double3/1
  FL controller via Eq. (15) with P control law v[k]/1(uck) -> Saturation5/1
  single2double3/1 -> FL controller via Eq. (15) with P control law v[k]/1(x1k_ref)
  single2double1/1 -> EHGO using Eq. (14)/1(yk)
  Rate Transition4/1 -> single2double4/1
  single2double4/1 -> EHGO using Eq. (14)/9(uck), uck/1
  Saturation5/1 -> Rate Transition4/1
  Constant28/1 -> single2double5/1
  single2double5/1 -> EHGO using Eq. (14)/2(Alpha1)
  Constant27/1 -> single2double6/1
  single2double6/1 -> EHGO using Eq. (14)/3(Alpha2)
  Constant26/1 -> single2double7/1
  single2double7/1 -> EHGO using Eq. (14)/4(Epsilon)
  Constant14/1 -> single2double8/1
  single2double8/1 -> EHGO using Eq. (14)/5(Kdpwm)
  Constant20/1 -> single2double9/1
  single2double9/1 -> EHGO using Eq. (14)/6(vdc)
  Constant8/1 -> single2double10/1
  single2double10/1 -> EHGO using Eq. (14)/7(L)
  Constant21/1 -> single2double11/1
  single2double11/1 -> EHGO using Eq. (14)/8(Ts)
  EHGO using Eq. (14)/1(zk_next) -> single2double2/1
  single2double2/1 -> Unit Delay/1
  Unit Delay/1 -> single2double12/1
  single2double12/1 -> FL controller via Eq. (15) with P control law v[k]/6(zk), EHGO using Eq. (14)/10(zk)
  Constant15/1 -> single2double13/1
  Constant19/1 -> single2double14/1
  Constant18/1 -> single2double15/1
  Constant17/1 -> single2double16/1
  single2double16/1 -> FL controller via Eq. (15) with P control law v[k]/2(Kdpwm)
  single2double15/1 -> FL controller via Eq. (15) with P control law v[k]/3(vdc)
  single2double14/1 -> FL controller via Eq. (15) with P control law v[k]/4(L)
  single2double13/1 -> FL controller via Eq. (15) with P control law v[k]/5(K1)
  Rate Transition3/1 -> Gain1/1
  G/1 -> Rate Transition3/1

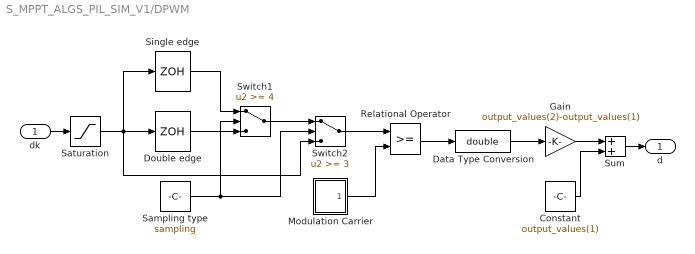
== system S_MPPT_ALGS_PIL_SIM_V1/DPWM ==
  dk : Inport
  Constant : Constant  Value=output_values(1)
  Data Type Conversion : DataTypeConversion  OutDataTypeStr=double  SaturateOnIntegerOverflow=on  RndMeth=Zero
  Double edge : ZeroOrderHold  SampleTime=si
  Gain : Gain  Gain=output_values(2)-output_values(1)  SaturateOnIntegerOverflow=on  OutDataTypeStr=Inherit: Same as input  ParamDataTypeStr=Inherit: Same as input
  Modulation Carrier : Subsystem  mask(Symmetric Triangle Generator){fc=fc, offset=mod(offset+.5, 1), range=input_limits}
      mask prompts: fc "Carrier frequency (Hz):"; offset "Carrier offset (p.u.):"; range "Signal range [min max]:"
      mask help: Generates a symmetrical triangular signal with output values between 0 and 1. The block forces the Simulink solver to output all tips of the signal. The output can therefore be used as a carrier signal for PWM.
      mask init:
      | if numel(fc)>1 || fc<=0,
      |   error('Carrier frequency must be a positive scalar.');
      | end
      | if numel(offset)>1 || offset<0 || offset>=1,
      |   error('Carrier offset must be a scalar in the interval [0; 1[.');
      | end
      | if numel(range)~=2,
      |   error('Signal range must be a two-element vector.')
      | end
      | if range(1)>=range(2),
      |   error('Signal range must be specified as [min max].')
      | end
      | 
      | carrier_t = [0 offset mod(1/2+offset, 1) 1]/fc;
      | carrier_v0 = 1-2*abs(offset-.5);
      | carrier_v = range(1)+[carrier_v0 0 1 carrier_v0]*diff(range);
      | [carrier_t, idx] = unique(carrier_t);
      | carrier_v = carrier_v(idx);
      | si = [.5 mod(offset, .5)]/fc;
      | 
      | L = length(carrier_t);
      | disp_seq_t = repmat(carrier_t(:),1,3) + ones(L,1)*[0,1,2]/fc;
      | disp_seq_v = repmat(carrier_v(:),1,3);
      mask Display: plot(disp_seq_t, disp_seq_v)
  Relational Operator : RelationalOperator  RndMeth=Nearest  InputSameDT=on
  Sampling type : Constant  Value=sampling
  Saturation : Saturate  UpperLimit=input_limits(2)  LowerLimit=input_limits(1)
  Single edge : ZeroOrderHold  SampleTime=[1 offset]/fc
  Sum : Sum  SaturateOnIntegerOverflow=on  InputSameDT=on  OutDataTypeStr=Inherit: Same as first input
  Switch1 : Switch  Threshold=4  SaturateOnIntegerOverflow=on  InputSameDT=on
  Switch2 : Switch  Threshold=3  SaturateOnIntegerOverflow=on  InputSameDT=on
  d : Outport
  wires:
  Data Type Conversion/1 -> Gain/1
  Constant/1 -> Sum/2
  Gain/1 -> Sum/1
  Sum/1 -> d/1
  Relational Operator/1 -> Data Type Conversion/1
  Switch2/1 -> Relational Operator/1
  Sampling type/1 -> Switch1/2, Switch2/2
  Single edge/1 -> Switch1/1
  Saturation/1 -> Double edge/1, Single edge/1, Switch2/3
  dk/1 -> Saturation/1
  Modulation Carrier/1(Out) -> Relational Operator/2
  Switch1/1 -> Switch2/1
  Double edge/1 -> Switch1/3

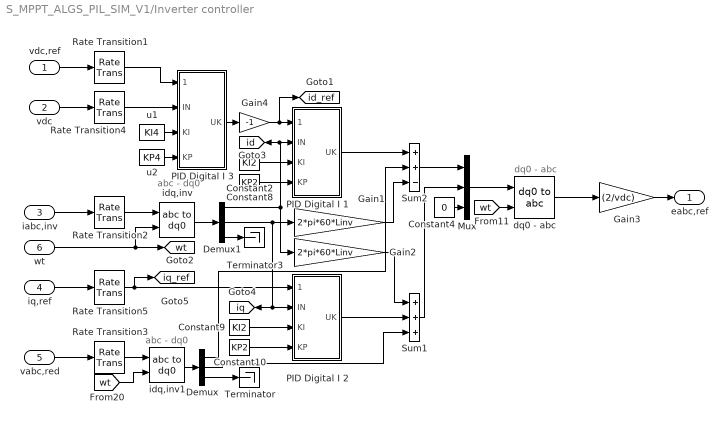
== system S_MPPT_ALGS_PIL_SIM_V1/Inverter controller ==
  note: dq0 - abc
  note: abc - dq0
  note: abc - dq0
  vdc,ref : Inport
  vdc : Inport  Port=2
  iabc,inv : Inport  Port=3
  iq,ref : Inport  Port=4
  vabc,red : Inport  Port=5
  wt : Inport  Port=6
  Constant10 : Constant  Value=KP2  SampleTime=Ts4
  Constant2 : Constant  Value=KI2  SampleTime=Ts4
  Constant4 : Constant  Value=0  SampleTime=Ts4
  Constant8 : Constant  Value=KP2  SampleTime=Ts4
  Constant9 : Constant  Value=KI2  SampleTime=Ts4
  Demux : Demux  Outputs=3
  Demux1 : Demux  Outputs=3
  Gain1 : Gain  Gain=2*pi*60*Linv
  Gain2 : Gain  Gain=2*pi*60*Linv
  Gain3 : Gain  Gain=(2/vdc)
  Gain4 : Gain  Gain=-1
  Mux : Mux  Inputs=3
  PID Digital I 1 : MATLAB Function  TreatAsAtomicUnit=on
  PID Digital I 2 : MATLAB Function  TreatAsAtomicUnit=on
  PID Digital I 3 : MATLAB Function  TreatAsAtomicUnit=on
  Rate Transition{1..5} (5 alike) : RateTransition  OutPortSampleTime=Ts4
  Sum1 : Sum  Inputs=+++
  Sum2 : Sum  Inputs=++-
  Terminator : Terminator
  Terminator3 : Terminator
  dq0 - abc : powerlib_meascontrol/Transformations/dq0 to abc  Alignment=90 degrees behind phase A axis
  idq,inv : powerlib_meascontrol/Transformations/abc to dq0  Alignment=90 degrees behind phase A axis
  idq,inv1 : powerlib_meascontrol/Transformations/abc to dq0  Alignment=90 degrees behind phase A axis
  u1 : Constant  Value=KI4  SampleTime=Ts4
  u2 : Constant  Value=KP4  SampleTime=Ts4
  eabc,ref : Outport
  tag scope: id=global, id_ref=global, iq=global, iq_ref=global, wt=global
  wires:
  vabc,red/1 -> Rate Transition3/1
  Rate Transition4/1 -> PID Digital I 3/2(IN)
  Demux/2 -> Sum1/3
  Demux1/2 -> PID Digital I 2/2(IN), [iq], Gain1/1
  PID Digital I 1/1(UK) -> Sum2/1
  Gain4/1 -> [id_ref], PID Digital I 1/1(IN_ref)
  Sum1/1 -> Mux/2
  Mux/1 -> dq0 - abc/1
  Constant4/1 -> Mux/3
  [wt] -> dq0 - abc/2
  Demux/3 -> Terminator/1
  Demux1/1 -> [id], PID Digital I 1/2(IN), Gain2/1
  Constant8/1 -> PID Digital I 1/4(KP)
  Rate Transition5/1 -> [iq_ref], PID Digital I 2/1(IN_ref)
  idq,inv1/1 -> Demux/1
  iq,ref/1 -> Rate Transition5/1
  idq,inv/1 -> Demux1/1
  Constant9/1 -> PID Digital I 2/3(KI)
  u1/1 -> PID Digital I 3/3(KI)
  vdc,ref/1 -> Rate Transition1/1
  Constant10/1 -> PID Digital I 2/4(KP)
  vdc/1 -> Rate Transition4/1
  Constant2/1 -> PID Digital I 1/3(KI)
  iabc,inv/1 -> Rate Transition2/1
  Rate Transition2/1 -> idq,inv/1
  Demux1/3 -> Terminator3/1
  Rate Transition3/1 -> idq,inv1/1
  u2/1 -> PID Digital I 3/4(KP)
  PID Digital I 2/1(UK) -> Sum1/2
  Sum2/1 -> Mux/1
  Demux/1 -> Sum2/2
  Gain2/1 -> Sum1/1
  Gain1/1 -> Sum2/3
  [wt] -> idq,inv1/2
  wt/1 -> [wt], idq,inv/2
  dq0 - abc/1 -> Gain3/1
  PID Digital I 3/1(UK) -> Gain4/1
  Rate Transition1/1 -> PID Digital I 3/1(IN_ref)
  Gain3/1 -> eabc,ref/1

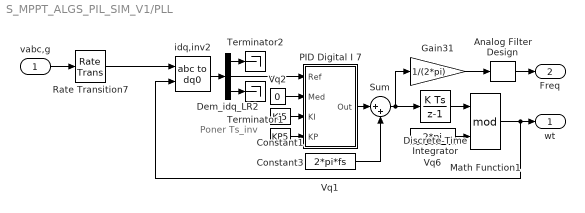
== system S_MPPT_ALGS_PIL_SIM_V1/PLL ==
  note: Poner Ts_inv
  vabc,g : Inport
  Analog Filter Design : dsparch4/Analog Filter Design  method=Butterworth  filttype=Lowpass  N=8  Wlo=4000  Whi=80  Rp=2  Rs=40
  Constant1 : Constant  Value=KI5  SampleTime=Ts_inv
  Constant3 : Constant  Value=KP5  SampleTime=Ts_inv
  Dem_idq_LR2 : Demux  Outputs=3
  Discrete-Time Integrator : DiscreteIntegrator  InitialConditionSetting=State (most efficient)  SampleTime=Ts_inv  ICPrevOutput=DiscIntNeverNeededParam  ICPrevScaledInput=DiscIntNeverNeededParam
  Gain31 : Gain  Gain=1/(2*pi)  OutMin=[0.1]
  Math Function1 : Math  Operator=mod  SaturateOnIntegerOverflow=on
  PID Digital I 7 : MATLAB Function  TreatAsAtomicUnit=on
  Rate Transition7 : RateTransition  OutPortSampleTime=Ts_inv
  Sum : Sum  Inputs=|++
  Terminator1 : Terminator
  Terminator2 : Terminator
  Vq1 : Constant  Value=2*pi*fs  SampleTime=Ts_inv
  Vq2 : Constant  Value=0
  Vq6 : Constant  Value=2*pi  SampleTime=Ts_inv
  idq,inv2 : powerlib_meascontrol/Transformations/abc to dq0  Alignment=90 degrees behind phase A axis
  wt : Outport
  Freq : Outport  Port=2
  wires:
  Gain31/1 -> Analog Filter Design/1
  vabc,g/1 -> Rate Transition7/1
  idq,inv2/1 -> Dem_idq_LR2/1
  Vq6/1 -> Math Function1/2
  Discrete-Time Integrator/1 -> Math Function1/1
  Math Function1/1 -> wt/1, idq,inv2/2
  Vq2/1 -> PID Digital I 7/2(Med)
  Dem_idq_LR2/2 -> PID Digital I 7/1(Ref)
  Sum/1 -> Gain31/1, Discrete-Time Integrator/1
  Vq1/1 -> Sum/2
  PID Digital I 7/1(Out) -> Sum/1
  Constant1/1 -> PID Digital I 7/3(KI)
  Constant3/1 -> PID Digital I 7/4(KP)
  Dem_idq_LR2/3 -> Terminator1/1
  Dem_idq_LR2/1 -> Terminator2/1
  Rate Transition7/1 -> idq,inv2/1
  Analog Filter Design/1 -> Freq/1

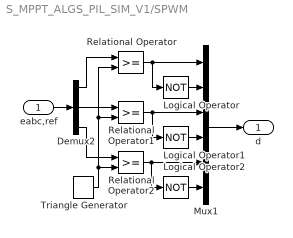
== system S_MPPT_ALGS_PIL_SIM_V1/SPWM ==
  eabc,ref : Inport
  Demux2 : Demux  Outputs=3
  Logical Operator : Logic  Operator=NOT  AllPortsSameDT=off  OutDataTypeStr=boolean
  Logical Operator1 : Logic  Operator=NOT  AllPortsSameDT=off  OutDataTypeStr=boolean
  Logical Operator2 : Logic  Operator=NOT  AllPortsSameDT=off  OutDataTypeStr=boolean
  Mux1 : Mux  Inputs=6
  Relational Operator : RelationalOperator  OutDataTypeStr=boolean  RndMeth=Simplest
  Relational Operator1 : RelationalOperator  OutDataTypeStr=boolean  RndMeth=Simplest
  Relational Operator2 : RelationalOperator  OutDataTypeStr=boolean  RndMeth=Simplest
  Triangle Generator : powerlib_meascontrol/Pulse & Signal Generators/Triangle Generator  Freq=Fc  Phase=0  Ts=Ts_inv
  d : Outport
  wires:
  Logical Operator/1 -> Mux1/2
  Demux2/1 -> Relational Operator/1
  Demux2/2 -> Relational Operator1/1
  Logical Operator1/1 -> Mux1/4
  Relational Operator2/1 -> Mux1/5, Logical Operator2/1
  Triangle Generator/1 -> Relational Operator2/2, Relational Operator1/2, Relational Operator/2
  Mux1/1 -> d/1
  Relational Operator/1 -> Logical Operator/1, Mux1/1
  Logical Operator2/1 -> Mux1/6
  Demux2/3 -> Relational Operator2/1
  Relational Operator1/1 -> Logical Operator1/1, Mux1/3
  eabc,ref/1 -> Demux2/1

== system S_MPPT_ALGS_PIL_SIM_V1/B Measumerents/Subsystem1 ==
  In1 : Inport
  In2 : Inport  Port=2
  MATLAB Function : MATLAB Function  TreatAsAtomicUnit=on
  Out1 : Outport
  wires:
  MATLAB Function/1(mse) -> Out1/1
  In1/1 -> MATLAB Function/1(Impp)
  In2/1 -> MATLAB Function/2(ipv)

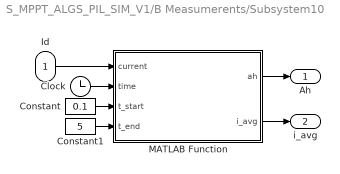
== system S_MPPT_ALGS_PIL_SIM_V1/B Measumerents/Subsystem10 ==
  Id : Inport
  Clock : Clock
  Constant : Constant  Value=0.1
  Constant1 : Constant  Value=5
  MATLAB Function : MATLAB Function  TreatAsAtomicUnit=on
  Ah : Outport
  i_avg : Outport  Port=2
  wires:
  MATLAB Function/1(ah) -> Ah/1
  Id/1 -> MATLAB Function/1(current)
  Clock/1 -> MATLAB Function/2(time)
  Constant/1 -> MATLAB Function/3(t_start)
  Constant1/1 -> MATLAB Function/4(t_end)
  MATLAB Function/2(i_avg) -> i_avg/1

== system S_MPPT_ALGS_PIL_SIM_V1/B Measumerents/Subsystem11 ==
  uc : Inport
  Clock : Clock
  Constant : Constant  Value=0.1
  Constant1 : Constant  Value=5
  MATLAB Function : MATLAB Function  TreatAsAtomicUnit=on
  uc_avg : Outport
  wires:
  MATLAB Function/1(uc_avg) -> uc_avg/1
  Constant/1 -> MATLAB Function/3(t_start)
  Constant1/1 -> MATLAB Function/4(t_end)
  uc/1 -> MATLAB Function/1(uc)
  Clock/1 -> MATLAB Function/2(time)

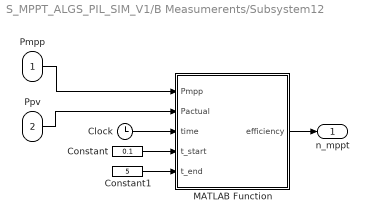
== system S_MPPT_ALGS_PIL_SIM_V1/B Measumerents/Subsystem12 ==
  Pmpp : Inport
  Ppv : Inport  Port=2
  Clock : Clock
  Constant : Constant  Value=0.1
  Constant1 : Constant  Value=5
  MATLAB Function : MATLAB Function  TreatAsAtomicUnit=on
  n_mppt : Outport
  wires:
  MATLAB Function/1(efficiency) -> n_mppt/1
  Constant/1 -> MATLAB Function/4(t_start)
  Constant1/1 -> MATLAB Function/5(t_end)
  Pmpp/1 -> MATLAB Function/1(Pmpp)
  Ppv/1 -> MATLAB Function/2(Pactual)
  Clock/1 -> MATLAB Function/3(time)

== system S_MPPT_ALGS_PIL_SIM_V1/B Measumerents/Subsystem14 ==
  PkW : Inport
  Clock : Clock
  Constant : Constant  Value=0.1
  Constant1 : Constant  Value=0.7
  MATLAB Function : MATLAB Function  TreatAsAtomicUnit=on
  wh : Outport
  Pw_avg : Outport  Port=2
  wires:
  MATLAB Function/1(energy_wh) -> wh/1
  PkW/1 -> MATLAB Function/1(power_kw)
  Clock/1 -> MATLAB Function/2(time)
  Constant/1 -> MATLAB Function/3(t_start)
  Constant1/1 -> MATLAB Function/4(t_end)
  MATLAB Function/2(power_avg) -> Pw_avg/1

== system S_MPPT_ALGS_PIL_SIM_V1/B Measumerents/Subsystem2 ==
  Pmpp : Inport
  Ppv : Inport  Port=2
  Clock : Clock
  Constant : Constant  Value=0.7
  Constant1 : Constant  Value=5.0
  MATLAB Function : MATLAB Function  TreatAsAtomicUnit=on
  nmppt : Outport
  wires:
  MATLAB Function/1(efficiency) -> nmppt/1
  Constant/1 -> MATLAB Function/4(t_start)
  Constant1/1 -> MATLAB Function/5(t_end)
  Pmpp/1 -> MATLAB Function/1(Pmpp)
  Ppv/1 -> MATLAB Function/2(Pactual)
  Clock/1 -> MATLAB Function/3(time)

== system S_MPPT_ALGS_PIL_SIM_V1/B Measumerents/Subsystem3 ==
  uc : Inport
  Clock : Clock
  Constant : Constant  Value=0.1
  Constant1 : Constant  Value=0.7
  MATLAB Function : MATLAB Function  TreatAsAtomicUnit=on
  uc_avg : Outport
  wires:
  MATLAB Function/1(uc_avg) -> uc_avg/1
  Constant/1 -> MATLAB Function/3(t_start)
  Constant1/1 -> MATLAB Function/4(t_end)
  uc/1 -> MATLAB Function/1(uc)
  Clock/1 -> MATLAB Function/2(time)

== system S_MPPT_ALGS_PIL_SIM_V1/B Measumerents/Subsystem4 ==
  uc : Inport
  Clock : Clock
  Constant : Constant  Value=0.7
  Constant1 : Constant  Value=5
  MATLAB Function : MATLAB Function  TreatAsAtomicUnit=on
  uc_avg : Outport
  wires:
  MATLAB Function/1(uc_avg) -> uc_avg/1
  Constant/1 -> MATLAB Function/3(t_start)
  Constant1/1 -> MATLAB Function/4(t_end)
  uc/1 -> MATLAB Function/1(uc)
  Clock/1 -> MATLAB Function/2(time)

== system S_MPPT_ALGS_PIL_SIM_V1/B Measumerents/Subsystem5 ==
  Pmpp : Inport
  Ppv : Inport  Port=2
  Clock : Clock
  Constant : Constant  Value=0.1
  Constant1 : Constant  Value=0.7
  MATLAB Function : MATLAB Function  TreatAsAtomicUnit=on
  nmppt : Outport
  wires:
  MATLAB Function/1(efficiency) -> nmppt/1
  Constant/1 -> MATLAB Function/4(t_start)
  Constant1/1 -> MATLAB Function/5(t_end)
  Pmpp/1 -> MATLAB Function/1(Pmpp)
  Ppv/1 -> MATLAB Function/2(Pactual)
  Clock/1 -> MATLAB Function/3(time)

== system S_MPPT_ALGS_PIL_SIM_V1/B Measumerents/Subsystem6 ==
  Id : Inport
  Clock : Clock
  Constant : Constant  Value=0.1
  Constant1 : Constant  Value=0.7
  MATLAB Function : MATLAB Function  TreatAsAtomicUnit=on
  Ah : Outport
  i_avg : Outport  Port=2
  wires:
  MATLAB Function/1(ah) -> Ah/1
  Id/1 -> MATLAB Function/1(current)
  Clock/1 -> MATLAB Function/2(time)
  Constant/1 -> MATLAB Function/3(t_start)
  Constant1/1 -> MATLAB Function/4(t_end)
  MATLAB Function/2(i_avg) -> i_avg/1

== system S_MPPT_ALGS_PIL_SIM_V1/B Measumerents/Subsystem7 ==
  Id : Inport
  Clock : Clock
  Constant : Constant  Value=0.7
  Constant1 : Constant  Value=5
  MATLAB Function : MATLAB Function  TreatAsAtomicUnit=on
  Ah : Outport
  i_avg : Outport  Port=2
  wires:
  MATLAB Function/1(ah) -> Ah/1
  Id/1 -> MATLAB Function/1(current)
  Clock/1 -> MATLAB Function/2(time)
  Constant/1 -> MATLAB Function/3(t_start)
  Constant1/1 -> MATLAB Function/4(t_end)
  MATLAB Function/2(i_avg) -> i_avg/1

== system S_MPPT_ALGS_PIL_SIM_V1/B Measumerents/Subsystem8 ==
  PkW : Inport
  Clock : Clock
  Constant : Constant  Value=0.7
  Constant1 : Constant  Value=5
  MATLAB Function : MATLAB Function  TreatAsAtomicUnit=on
  wh : Outport
  Pw_avg : Outport  Port=2
  wires:
  MATLAB Function/1(energy_wh) -> wh/1
  PkW/1 -> MATLAB Function/1(power_kw)
  Clock/1 -> MATLAB Function/2(time)
  Constant/1 -> MATLAB Function/3(t_start)
  Constant1/1 -> MATLAB Function/4(t_end)
  MATLAB Function/2(power_avg) -> Pw_avg/1

== system S_MPPT_ALGS_PIL_SIM_V1/B Measumerents/Subsystem9 ==
  PkW : Inport
  Clock : Clock
  Constant : Constant  Value=0.1
  Constant1 : Constant  Value=5
  MATLAB Function : MATLAB Function  TreatAsAtomicUnit=on
  wh : Outport
  Pw_avg : Outport  Port=2
  wires:
  MATLAB Function/1(energy_wh) -> wh/1
  PkW/1 -> MATLAB Function/1(power_kw)
  Clock/1 -> MATLAB Function/2(time)
  Constant/1 -> MATLAB Function/3(t_start)
  Constant1/1 -> MATLAB Function/4(t_end)
  MATLAB Function/2(power_avg) -> Pw_avg/1

== system S_MPPT_ALGS_PIL_SIM_V1/DPWM/Modulation Carrier ==
  Clock : Clock
  Fcn : Fcn  Expr=u*fc-offset
  Lookup Table : Lookup  InputValues=[0 .5 1]  Table=[range(1) range(2) range(1)]  LookUpMeth=Interpolation-Use End Values
  Rounding Function : Rounding
  Subtract : Sum  Inputs=+-
  Unit Delay : UnitDelay  SampleTime=si
  Out : Outport
  wires:
  Lookup Table/1 -> Out/1
  Subtract/1 -> Lookup Table/1
  Rounding Function/1 -> Subtract/2
  Fcn/1 -> Rounding Function/1, Subtract/1
  Clock/1 -> Fcn/1
  Unit Delay/1 -> Unit Delay/1

== matlab function S_MPPT_ALGS_PIL_SIM_V1/B Measumerents/Subsystem2/MATLAB Function ==
  data: efficiency output; Pmpp input; Pactual input; time input; t_start input; t_end input

function efficiency = n_mppt(Pmpp, Pactual, time, t_start, t_end)
%#codegen
% Calcula la eficiencia acumulada de un MPPT en porcentaje
% limitando Pactual para que no exceda Pmpp.
% Acumula solo dentro del intervalo de tiempo [t_start, t_end].
%
% Entradas:
%   Pmpp     : potencia teórica máxima (kW)
%   Pactual  : potencia medida real (kW)
%   time     : tiempo actual (segundos)
%   t_start  : inicio de acumulación
%   t_end    : fin de acumulación
%
% Salida:
%   efficiency : eficiencia acumulada (%), limitada a 100

% Variables persistentes
persistent total_Pmpp total_Pactual started

% Inicialización al primer uso
if isempty(total_Pmpp)
    total_Pmpp = 0;
    total_Pactual = 0;
    started = false;
end

% Acumular solo dentro del intervalo [t_start, t_end]
if time >= t_start && time <= t_end
    if ~started
        started = true;
    end

    % Limitar Pactual para evitar que exceda Pmpp
    %Pactual_limited = min(Pactual, Pmpp);
     
    % No Limitar Pactual 
    Pactual_limited = Pactual;

    % Acumulación
    total_Pmpp = total_Pmpp + Pmpp;
    total_Pactual = total_Pactual + Pactual_limited;
end

% Cálculo de eficiencia acumulada
if total_Pmpp < 1e-6
    efficiency = 0;
else
    efficiency = min((total_Pactual / total_Pmpp) * 100, 100);
end
end

== matlab function S_MPPT_ALGS_PIL_SIM_V1/Inverter controller/PID Digital I 1 ==
  data: IN_ref input; UK output; IN input; KI input; KP input
function UK = fcn(IN_ref, IN, KI, KP)

 %Valores iniciales de las conStantes del controlador
 persistent  ek uk
 persistent  ek_1 uk_1
 if isempty(ek)
    ek =0;
    uk =0;
    ek_1 =0;
    uk_1 =0;
 end
ek=IN_ref-IN;
uk=ek*(KP+KI)-ek_1*KP+uk_1;
if(uk>1000)
    uk=1000;
end
if(uk<-1000)
    uk=-1000;
end
ek_1=ek;
uk_1=uk;
UK=uk;
end

== matlab function S_MPPT_ALGS_PIL_SIM_V1/Inverter controller/PID Digital I 2 ==
  data: IN_ref input; UK output; IN input; KI input; KP input
function UK = fcn(IN_ref, IN, KI, KP)

 %Valores iniciales de las conStantes del controlador
 persistent  ek uk
 persistent  ek_1 uk_1
 if isempty(ek)
    ek =0;
    uk =0;
    ek_1 =0;
    uk_1 =0;
 end
ek=IN_ref-IN;
uk=ek*(KP+KI)-ek_1*KP+uk_1;
if(uk>1000)
    uk=1000;
end
if(uk<-1000)
    uk=-1000;
end
ek_1=ek;
uk_1=uk;
UK=uk;
end

== matlab function S_MPPT_ALGS_PIL_SIM_V1/Inverter controller/PID Digital I 3 ==
  data: IN_ref input; UK output; IN input; KI input; KP input
function UK = fcn(IN_ref, IN, KI, KP)

 %Valores iniciales de las conStantes del controlador
 persistent  ek uk
 persistent  ek_1 uk_1
 if isempty(ek)
    ek =0;
    uk =0;
    ek_1 =0;
    uk_1 =0;
 end
ek=IN_ref-IN;
uk=ek*(KP+KI)-ek_1*KP+uk_1;
if(uk>60)
    uk=60;
end
if(uk<-60)
    uk=-60;
end
ek_1=ek;
uk_1=uk;
UK=uk;
end

== matlab function S_MPPT_ALGS_PIL_SIM_V1/PLL/PID Digital I 7 ==
  data: Ref input; Out output; Med input; KI input; KP input
function Out = fcn(Ref, Med, KI, KP)

 %Valores iniciales de las conStantes del controlador
 persistent  ek uk
 persistent  ek_1 uk_1
 if isempty(ek)
    ek =0;
    uk =0;
    ek_1 =0;
    uk_1 =0;
 end
ek=Ref-Med;
%uk=ek*(KP+KI)-ek_1*KP+uk_1;
uk=KP*ek+KI*ek+KI*ek_1;
ek_1=ek;
uk_1=uk;
Out=uk;
end

== matlab function S_MPPT_ALGS_PIL_SIM_V1/Cont Real Est1/PID Digital I 3 ==
  data: x1k_ref input; uck output; x1k input; KI input; KP input
function uck = fcn(x1k_ref, x1k, KI, KP)

 %Valores iniciales de las conStantes del controlador
 persistent  ek uk
 persistent  ek_1 uk_1
 if isempty(ek)
    ek =0;
    uk =0;
    ek_1 =0;
    uk_1 =0;
 end
ek=x1k_ref-x1k;
uk=ek*(KP+KI)-ek_1*KP+uk_1;
%uk=KP*ek+KI*ek+KI*ek_1;
% if(uk>(1*65535))
%     uk=1*65535;
% end
% if(uk<0)
%     uk=0;
% end
ek_1=ek;
uk_1=uk;
uck=uk;
end

== matlab function S_MPPT_ALGS_PIL_SIM_V1/Cont Real Est2/EHGO using Eq. (14) ==
  data: yk input; Alpha1 input; Alpha2 input; Epsilon input; Kdpwm input; vdc input; L input; Ts input; uck input; zk input; zk_next output
function zk_next = fcn(yk, Alpha1, Alpha2, Epsilon, Kdpwm, vdc, L, Ts, uck, zk)
zk_next = zeros(2,1);
zk_next(1) = zk(1) + Ts*(zk(2)+((Kdpwm/L)*vdc)*uck+ (Alpha1/(Epsilon*Ts))*(yk-zk(1)));
zk_next(2) = zk(2) + Ts*((Alpha2/(Epsilon^2*Ts^2))*(yk-zk(1)));

== matlab function S_MPPT_ALGS_PIL_SIM_V1/B Measumerents/Subsystem5/MATLAB Function ==
  data: efficiency output; Pmpp input; Pactual input; time input; t_start input; t_end input

function efficiency = n_mppt(Pmpp, Pactual, time, t_start, t_end)
%#codegen
% Calcula la eficiencia acumulada de un MPPT en porcentaje
% limitando Pactual para que no exceda Pmpp.
% Acumula solo dentro del intervalo de tiempo [t_start, t_end].
%
% Entradas:
%   Pmpp     : potencia teórica máxima (kW)
%   Pactual  : potencia medida real (kW)
%   time     : tiempo actual (segundos)
%   t_start  : inicio de acumulación
%   t_end    : fin de acumulación
%
% Salida:
%   efficiency : eficiencia acumulada (%), limitada a 100

% Variables persistentes
persistent total_Pmpp total_Pactual started

% Inicialización al primer uso
if isempty(total_Pmpp)
    total_Pmpp = 0;
    total_Pactual = 0;
    started = false;
end

% Acumular solo dentro del intervalo [t_start, t_end]
if time >= t_start && time <= t_end
    if ~started
        started = true;
    end

    % Limitar Pactual para evitar que exceda Pmpp
    %Pactual_limited = min(Pactual, Pmpp);
     
    % No Limitar Pactual 
    Pactual_limited = Pactual;

    % Acumulación
    total_Pmpp = total_Pmpp + Pmpp;
    total_Pactual = total_Pactual + Pactual_limited;
end

% Cálculo de eficiencia acumulada
if total_Pmpp < 1e-6
    efficiency = 0;
else
    efficiency = min((total_Pactual / total_Pmpp) * 100, 100);
end
end

== matlab function S_MPPT_ALGS_PIL_SIM_V1/Cont Real Est2/FL controller via Eq. (15) with P control law v[k] ==
  data: x1k_ref input; Kdpwm input; vdc input; L input; K1 input; uck output; zk input
function uck = fcn(x1k_ref, Kdpwm, vdc, L, K1, zk)
uck=(L/(Kdpwm*vdc))*(-zk(2)+(-K1*(zk(1)-x1k_ref)));

== matlab function S_MPPT_ALGS_PIL_SIM_V1/B Measumerents/Subsystem1/MATLAB Function ==
  data: mse output; Impp input; ipv input
function mse = mse_tracking(Impp, ipv)
%#codegen
% Calcula el error cuadrático medio acumulado entre la corriente de referencia (Impp)
% y la corriente real del arreglo fotovoltaico (ipv)
% Entradas:
%   Impp: corriente de referencia (punto de máxima potencia)
%   ipv: corriente medida real del arreglo PV
% Salida:
%   mse: error cuadrático medio acumulado

% Variables persistentes para acumulación
persistent sum_squared_error sample_count

% Inicialización al primer uso
if isempty(sum_squared_error)
    sum_squared_error = 0;
    sample_count = 0;
end

% Cálculo del error y actualización
error = Impp - ipv;
sum_squared_error = sum_squared_error + error^2;
sample_count = sample_count + 1;

% Cálculo del MSE acumulado
if sample_count == 0
    mse = 0;
else
    mse = sum_squared_error / sample_count;
end
end

== matlab function S_MPPT_ALGS_PIL_SIM_V1/Cont Real Est/PID Digital I 2 ==
  data: x1k_Ref input; x1k input; x2k input; uck output; Ki input; K1 input; K2 input; Ts input
function uck = fcn(x1k_Ref, x1k, x2k, Ki, K1, K2, Ts)
    % Retroalimentación de estados con acción integral
    
    % Variables persistentes para mantener el estado entre llamadas
    persistent ek Acc_Int Acc_Int_1 uk
    
    if isempty(ek)
        ek = 0;
        Acc_Int = 0;
        Acc_Int_1 = 0;
        uk = 0;
    end

    % Cálculo del error
    ek = x1k_Ref - x1k;

    % Acción integral
    Acc_Int = Ki * ek * Ts + Acc_Int_1;
    Acc_Int_1 = Acc_Int;

    % Ley de control: acción integral menos retroalimentación de estados
    uk = Acc_Int - (K1 * x1k + K2 * x2k);

%     % Saturación (opcional)
%     uk = min(max(uk, 0), 65535);

    % Salida del controlador
    uck = uk;
end
